simulink model "Q5"  (R2016a)
settings: Solver=VariableStepAuto  StartTime=0.0  StopTime=stop  RelTol=1e-10
values from neighbouring files (symbols this model uses):
  beta = 0.001    [e_13.m]    (also in e_8.m = 1; e_9.m; lab3.m; lab3_1.m = 1)
  g = 9.8    [e_13.m]    (also in e_8.m; e_9.m; lab3.m; lab3_1.m)
  J = ((M*L^2)/3) + (m * l(n)^2)    [e_12.m]    (also in e_13.m = M*L^2/3+m_s*l^2; e_8.m = 0.0445; e_9.m = ((M*L^2)/3) + (m * l^2); lab3.m = M*L^2/3+m_s*l^2)
  k = 0.35    [e_13.m]    (also in e_8.m = 3; e_9.m; lab3.m; lab3_1.m = 3)
  l = l_c_nl(n)    [e_10.m]    (also in e_11.m = l_c(2); e_12.m = l_c; e_13.m = l_c(1); e_8.m = 0.4)
  L = 0.25    [e_13.m]    (also in e_8.m = 0.5; e_9.m; lab3.m; lab3_1.m = 0.5)
  m = 0.2    [e_8.m]    (also in e_9.m = m_c; lab3.m = m_c; lab3_1.m; lab3_2.m = m_c)
  M = 0.1    [e_13.m]    (also in e_8.m = 0.15; e_9.m; lab3.m; lab3_1.m = 0.15)
  T = T_v(n)    [e_11.m]    (also in e_13.m = 0; e_8.m = 0; e_9.m = 0; lab3.m = 0)
  x0 = [pi/4 0]    [e_13.m]    (also in e_8.m = vec_prop(:,n); e_9.m; lab3.m; lab3_1.m = [0 pi/4])
settings Model: Creator=ricar  LastModifiedBy=ricar

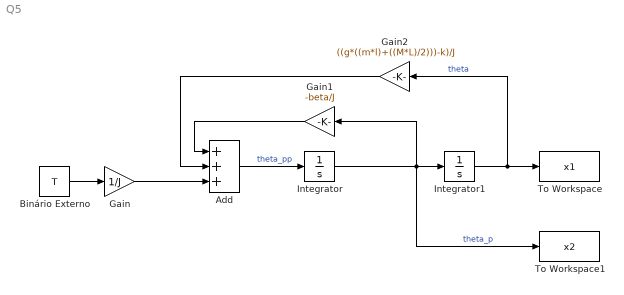
== system Q5 ==
  Add : Sum  Inputs=+++
  Binário Externo : Constant  Value=T
  Gain : Gain  Gain=1/J
  Gain1 : Gain  Gain=-beta/J
  Gain2 : Gain  Gain=((g*((m*l)+((M*L)/2)))-k)/J
  Integrator : Integrator  InitialCondition=x0(2)
  Integrator1 : Integrator  InitialCondition=x0(1)
  To Workspace : ToWorkspace  VariableName=x1  SampleTime=-1
  To Workspace1 : ToWorkspace  VariableName=x2  SampleTime=-1
  wires:
  Binário Externo/1 -> Gain/1
  Gain/1 -> Add/3
  Add/1 -> Integrator/1  "theta_pp"
  Integrator/1 -> Gain1/1, To Workspace1/1, Integrator1/1  "theta_p"
  Integrator1/1 -> Gain2/1, To Workspace/1  "theta"
  Gain1/1 -> Add/1
  Gain2/1 -> Add/2
